simulink model "IMU_dsPIC_30f4012_ComplementaryFilter_20Mips"  (Simulink 7.1)
settings: Solver=FixedStepDiscrete  StartTime=0.0  StopTime=10.0  FixedStep=0.001  RelTol=1e-3
PreLoadFcn:
  | Script_Kalman
undefined symbols (not defined in the file or in its folder): DiscIntNeverNeededParam, gaind, polesd, zerosd
libraries: simulink x10, dsPICdrivers x10
CloseFcn:
  | rtwprivate ssgencode ModelCloseRequest Autopilote_30f4012
settings Model: Creator=Lubin  LastModifiedBy=Lubin
settings OptimizationCC: InlineParams=on  OptimizeModelRefInitCode=on  LifeSpan=1
settings DebuggingCC: SaveWithParameterizedLinksMsg=none  MultiTaskCondExecSysMsg=warning  MultiTaskRateTransMsg=warning
settings HardwareCC: ProdBitPerInt=16  ProdEndianess=LittleEndian  ProdWordSize=16  ProdHWDeviceType=16-bit Generic
settings RTWCC: SystemTargetFile=dspic.tlc  TemplateMakefile=dspic_pic30_gcc.tmf  PostCodeGenCommand=dsPIC_Compile()  Description=Embedded Target for Microchip dsPIC (real-time)  GenerateReport=on  ProcessScript=dspic_make_rtw_hook  IncludeHyperlinkInReport=on  LaunchReport=on  GenerateTraceInfo=on  GenerateTraceReport=on  GenerateTraceReportSl=on  GenerateTraceReportSf=on  GenerateTraceReportEml=on
settings CodeAppCC: IgnoreCustomStorageClasses=off
settings STFCustomTargetCC: ModelReferenceCompliant=off  IncludeMdlTerminateFcn=off  CombineOutputUpdateFcns=on  SuppressErrorStatus=on  ERTCustomFileBanners=on  SupportContinuousTime=off  SupportNonInlinedSFcns=off  SystemTargetFile=dspic.tlc
settings ERTTargetCC: ModelReferenceCompliant=off  CompOptLevelCompliant=off  IncludeMdlTerminateFcn=off  SuppressErrorStatus=on  ERTFirstTimeCompliant=off  ModelStepFunctionPrototypeControlCompliant=off  ExtModeMexFile=ext_serial_win32_comm  InlinedParameterPlacement=NonHierarchical  ERTSrcFileBannerTemplate=dsPIC_code_template.cgt  ERTHdrFileBannerTemplate=dsPIC_code_template.cgt  ERTDataSrcFileTemplate=dsPIC_code_template.cgt  ERTDataHdrFileTemplate=dsPIC_code_template.cgt  ERTCustomFileTemplate=dsPIC_main.tlc
settings CustomProperty: DataType=string  Value=C:\PROGRA~1\MATLAB\R2008a\bin\win32\gmake

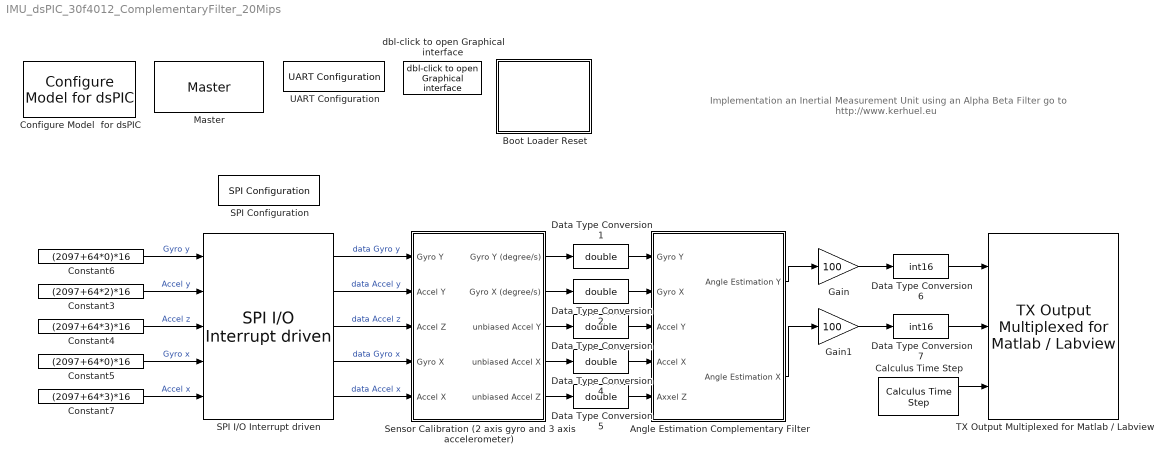
== system IMU_dsPIC_30f4012_ComplementaryFilter_20Mips ==
  note: Implementation an Inertial Measurement Unit using an Alpha Beta Filter
      | go to http://www.kerhuel.eu
  Angle Estimation Complementary Filter : Subsystem
  Boot Loader Reset : Subsystem  AncestorBlock=dsPICdrivers/OTHERS/TinyBld Reset
      mask Display: fprintf('TinyBld\nReset')
  Calculus Time Step : dsPICdrivers/OTHERS/Calculus Time Step  Tag=dsPIC_CalculusTimeStep  SampleTime=-1  PR1chk=on
  Configure Model  for dsPIC : dsPICdrivers/Simulink Configuration/Configure Model  for dsPIC
  Constant3 : Constant  Value=(2097+64*2)*16  VectorParams1D=off  OutDataTypeMode=uint16  OutDataType=sfix(16)  OutScaling=2^0  OutDataTypeStr=uint16  SampleTime=-1
  Constant4 : Constant  Value=(2097+64*3)*16  VectorParams1D=off  OutDataTypeMode=uint16  OutDataType=sfix(16)  OutScaling=2^0  OutDataTypeStr=uint16  SampleTime=-1
  Constant5 : Constant  Value=(2097+64*0)*16  VectorParams1D=off  OutDataTypeMode=uint16  OutDataType=sfix(16)  OutScaling=2^0  OutDataTypeStr=uint16  SampleTime=-1
  Constant6 : Constant  Value=(2097+64*0)*16  VectorParams1D=off  OutDataTypeMode=uint16  OutDataType=sfix(16)  OutScaling=2^0  OutDataTypeStr=uint16  SampleTime=-1
  Constant7 : Constant  Value=(2097+64*3)*16  VectorParams1D=off  OutDataTypeMode=uint16  OutDataType=sfix(16)  OutScaling=2^0  OutDataTypeStr=uint16  SampleTime=-1
  Data Type Conversion{,1..2,4..5} (5 alike) : DataTypeConversion  OutDataTypeMode=double  OutDataType=sfix(16)  OutScaling=2^0  OutDataTypeStr=double
  Data Type Conversion6 : DataTypeConversion  OutDataTypeMode=int16  OutDataType=sfix(16)  OutScaling=2^0  OutDataTypeStr=int16
  Data Type Conversion7 : DataTypeConversion  OutDataTypeMode=int16  OutDataType=sfix(16)  OutScaling=2^0  OutDataTypeStr=int16
  Gain : Gain  Gain=100  ParameterDataType=sfix(16)  ParameterScaling=2^0  OutDataType=sfix(16)  OutScaling=2^0
  Gain1 : Gain  Gain=100  ParameterDataType=sfix(16)  ParameterScaling=2^0  OutDataType=sfix(16)  OutScaling=2^0
  Master : dsPICdrivers/Master  Tag=dsPIC_MASTER  Priority=1  TimeStepType=Timer1  picType=30f4012  fcy=20e6  Quartz_33f=5e6  PLLActive_33f=off  fcyDesired_33f=0  tmr1="[1  19999  0]"  tmr1Info="Time Step : 0.001  ;   Error : 0%  PR1=19999"  tmr2345="[0  0  0  0]"  tmr2345cfg=[-1 -1 -1 -1]  IOautoConf=on  typePort="[ 0   0   0   0   0   0   0   0   0   0   0   0   0   0   0   0   0   0   0   0   0   0   0   0   0   0   0   0   0   0   0   0   0   0   0   0   0   0   0   0   0   0   0   0   0   5   4   0   0   0   0   0   0   0   0   0   0   0   0   0   0   0   0   0   0   0   0  21   0  21   0   0  17   0   0   0   0   0   0   0   0   0   0   0   0   0   0   0   0   0   0   0   0   0   0   0   0   0   0   0   0   0   0   0   0   0   0   0   0   0   0   0 ]"  TRIS="[ 65535  65535  65535  65535  65495  65535  65535 ]"  ADPCFG=0  MasterBusyPort=None  MasterOverloadPort=None  FOSC=XT_PLL8  TempProtection_33f=TEMP_ON  FPBOR=PBOR_OFF  PWRT=PWRT_4  MCLR=MCLR_DIS  PowerSave=off
  SPI Configuration : dsPICdrivers/SPI PORT/SPI Configuration  Tag=dsPIC_config_SPI  Priority=2  ConfigurationTime=At boot time (only once)  OrderingInOutPopup=None  SampleTime=-1  Frame_Enable=0  Frame_Sync=0  SPI=1  MODE=MASTER  USER_SCALER=96  StartEnable=Enable  SDO_EN=on  DATA_LENGTH=16 bits  SS_EN=off  SMP=Middle of bit  CKP=high  CKE=Idle to Active  Status="Mode 1  -    Fsck= Not Available"
  SPI I/O Interrupt driven : dsPICdrivers/SPI PORT/SPI I//O Interrupt driven  Tag=dsPIC_SPI_IO_Interrupt  SPI=1  nbrTrame=5  mode=read once - interrupt re-enable after block execution  Disable=on  DATA_LENGTH=16 bits  OrderingInOutPopup=None  SampleTime=.001  T1CSL=E5  T1CSH=None  T2CSL=E5  T2CSH=None  T3CSL=E5  T3CSH=None  T4CSL=E3  T4CSH=None  T5CSL=E3  T5CSH=None  T6CSL=None  T6CSH=None  T7CSL=None  T7CSH=None  T8CSL=None  T8CSH=None  T9CSL=None  T9CSH=None  T10CSL=None  T10CSH=None  T11CSL=None  T11CSH=None  T12CSL=None  T12CSH=None  T13CSL=None  T13CSH=None  T14CSL=None  T14CSH=None  T15CSL=None  T15CSH=None
  Sensor Calibration (2 axis gyro and 3 axis accelerometer) : Subsystem
  TX Output Multiplexed for Matlab / Labview : dsPICdrivers/Serial PORT/TX Output Multiplexed for Matlab // Labview  Tag=dsPIC_TX_Multiplexed  Priority=5  UART=1  CleverSpreadingChk=on  CleverSpreading=1  CHANNEL=[0 1 2]  CHANNELBLOCKED=[]  CHANNELBLOCKED_BITEWISE=0  Status=OK
  UART Configuration : dsPICdrivers/Serial PORT/UART Configuration  Tag=dsPIC_config_UART  Priority=2  UART=1  proposed_BAUD=115200  ALT_TX_RX=on  InterruptTxWhen=When Transmit Buffer is empty  TXInterruptPri=1  TxBufferSize=32  TXEN=on  InterruptRxWhen=When Receive Buffer is full (contain 4 characters)  RXInterruptPri=1  RxBufferSize=32  BAUD=115200  UxBRG=10  Info="UxBRG = 10   ||  Real Baud : 113636   ||  % error : -1.3573  ||  max 11.3636 Bytes / Step"  RealBaud=0
  dbl-click to open Graphical interface : dsPICdrivers/Serial PORT/dbl-click to open Graphical interface  SystemSampleTime=-1  Nothing=0
  wires:
  Constant6/1 -> SPI I/O Interrupt driven/1  "Gyro y"
  Constant3/1 -> SPI I/O Interrupt driven/2  "Accel y"
  Constant4/1 -> SPI I/O Interrupt driven/3  "Accel z"
  Constant5/1 -> SPI I/O Interrupt driven/4  "Gyro x"
  Constant7/1 -> SPI I/O Interrupt driven/5  "Accel x"
  Gain/1 -> Data Type Conversion6/1
  Gain1/1 -> Data Type Conversion7/1
  Data Type Conversion6/1 -> TX Output Multiplexed for Matlab / Labview/1
  Data Type Conversion7/1 -> TX Output Multiplexed for Matlab / Labview/2
  Calculus Time Step/1 -> TX Output Multiplexed for Matlab / Labview/3
  SPI I/O Interrupt driven/1 -> Sensor Calibration (2 axis gyro and 3 axis accelerometer)/1(Gyro Y)  "data Gyro y"
  SPI I/O Interrupt driven/2 -> Sensor Calibration (2 axis gyro and 3 axis accelerometer)/2(Accel Y)  "data Accel y"
  SPI I/O Interrupt driven/3 -> Sensor Calibration (2 axis gyro and 3 axis accelerometer)/3(Accel Z)  "data Accel z"
  SPI I/O Interrupt driven/4 -> Sensor Calibration (2 axis gyro and 3 axis accelerometer)/4(Gyro X)  "data Gyro x"
  SPI I/O Interrupt driven/5 -> Sensor Calibration (2 axis gyro and 3 axis accelerometer)/5(Accel X)  "data Accel x"
  Data Type Conversion1/1 -> Angle Estimation Complementary Filter/1("Gyro Y ")
  Data Type Conversion2/1 -> Angle Estimation Complementary Filter/2(Gyro X)
  Data Type Conversion/1 -> Angle Estimation Complementary Filter/3(Accel Y)
  Data Type Conversion4/1 -> Angle Estimation Complementary Filter/4(Accel X)
  Data Type Conversion5/1 -> Angle Estimation Complementary Filter/5(Axxel Z)
  Sensor Calibration (2 axis gyro and 3 axis accelerometer)/1(Gyro Y (degree/s)) -> Data Type Conversion1/1
  Sensor Calibration (2 axis gyro and 3 axis accelerometer)/2(Gyro X (degree/s)) -> Data Type Conversion2/1
  Angle Estimation Complementary Filter/1(Angle Estimation Y) -> Gain/1
  Angle Estimation Complementary Filter/2(Angle Estimation X) -> Gain1/1
  Sensor Calibration (2 axis gyro and 3 axis accelerometer)/3(unbiased Accel Y) -> Data Type Conversion/1
  Sensor Calibration (2 axis gyro and 3 axis accelerometer)/4(unbiased Accel X) -> Data Type Conversion4/1
  Sensor Calibration (2 axis gyro and 3 axis accelerometer)/5(unbiased Accel Z) -> Data Type Conversion5/1

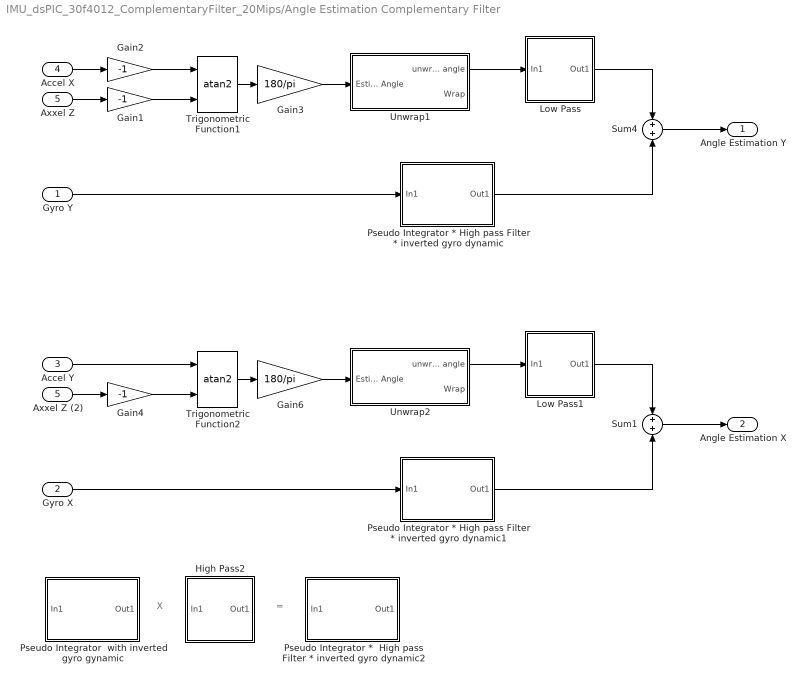
== system IMU_dsPIC_30f4012_ComplementaryFilter_20Mips/Angle Estimation Complementary Filter ==
  note: =
  note: X
  "Gyro Y " : Inport
  Gyro X : Inport  Port=2
  Accel Y : Inport  Port=3
  Accel X : Inport  Port=4
  Axxel Z : Inport  Port=5
  Axxel Z (2) : InportShadow  Port=5  LatchByCopyingInsideSignal=off
  Gain1 : Gain  Gain=-1  ParameterDataType=sfix(16)  ParameterScaling=2^0  OutDataType=sfix(16)  OutScaling=2^0
  Gain2 : Gain  Gain=-1  ParameterDataType=sfix(16)  ParameterScaling=2^0  OutDataType=sfix(16)  OutScaling=2^0
  Gain3 : Gain  Gain=180/pi  ParameterDataType=sfix(16)  ParameterScaling=2^0  OutDataTypeMode=Specify via dialog  OutDataType=float('double')  OutDataTypeStr=float('double')
  Gain4 : Gain  Gain=-1  ParameterDataType=sfix(16)  ParameterScaling=2^0  OutDataType=sfix(16)  OutScaling=2^0
  Gain6 : Gain  Gain=180/pi  ParameterDataType=sfix(16)  ParameterScaling=2^0  OutDataTypeMode=Specify via dialog  OutDataType=float('double')  OutDataTypeStr=float('double')
  High Pass2 : Subsystem  mask(DiscretizedZeroPole){Zeros=[0], Poles=[-.5], Gain=1, AbsTol=auto, SampleTime=.001, method=tustin, Wc=1}
      mask prompts: Zeros "Zeros (enter in s-main:)"; Poles "Poles (enter in s-domain:)"; Gain "Gain (enter in s-domain:)"; AbsTol "Absolute tolerance:"; SampleTime "Sample time:"; Wc "Critical Frequency (Hz):"
      mask help: Continuous mask uses c2d to transform parameters onto the Discrete Zero-Pole block inside.
      mask init:
      | st=SampleTime;
      | if length(st)>1
      |     st=SampleTime(1);
      | end
      | if(st>0)
      |     [zerosd,polesd,gaind] = sldiscutil('disczpk', {st,method,Wc,Zeros,Poles,Gain});
      | end	
      | s = get_param(gcb,'maskvalues');
      | zeross = s{1};
      | poless = s{2};
      | gainss = s{3};
      | %zerosc = eval(zeross);
      | %polesc = eval(poless);
      | %gainsc = eval(gainss);
      | sldiscutil('initzpkmask', st);
      | if(st==0)
      | set_param([gcb '/Zero Pole'], 'AbsoluteTolerance', AbsTol);
      | end
      mask StyleString: edit,edit,edit,edit,edit,popup(zoh|foh|tustin|prewarp|matched),edit
      mask CallbackString: |||||hidecrit|
      mask Display:
      | droots(zeross,poless,gainss)
      | text( 0.5, 1.0, method, 'verticalAlignment','top')
  Low Pass : Subsystem  mask(DiscretizedZeroPole){Zeros=[], Poles=[-.5], Gain=.5, AbsTol=auto, SampleTime=.001, method=tustin, Wc=1}
      mask prompts: Zeros "Zeros (enter in s-main:)"; Poles "Poles (enter in s-domain:)"; Gain "Gain (enter in s-domain:)"; AbsTol "Absolute tolerance:"; SampleTime "Sample time:"; Wc "Critical Frequency (Hz):"
      mask help: Continuous mask uses c2d to transform parameters onto the Discrete Zero-Pole block inside.
      mask init: same as IMU_dsPIC_30f4012_ComplementaryFilter_20Mips/Angle Estimation Complementary Filter/High Pass2
      mask StyleString: edit,edit,edit,edit,edit,popup(zoh|foh|tustin|prewarp|matched),edit
      mask CallbackString: |||||hidecrit|
      mask Display:
      | droots(zeross,poless,gainss)
      | text( 0.5, 1.0, method, 'verticalAlignment','top')
  Low Pass1 : Subsystem  mask(DiscretizedZeroPole){Zeros=[], Poles=[-.5], Gain=.5, AbsTol=auto, SampleTime=.001, method=tustin, Wc=1}
      mask prompts: Zeros "Zeros (enter in s-main:)"; Poles "Poles (enter in s-domain:)"; Gain "Gain (enter in s-domain:)"; AbsTol "Absolute tolerance:"; SampleTime "Sample time:"; Wc "Critical Frequency (Hz):"
      mask help: Continuous mask uses c2d to transform parameters onto the Discrete Zero-Pole block inside.
      mask init: same as IMU_dsPIC_30f4012_ComplementaryFilter_20Mips/Angle Estimation Complementary Filter/High Pass2
      mask StyleString: edit,edit,edit,edit,edit,popup(zoh|foh|tustin|prewarp|matched),edit
      mask CallbackString: |||||hidecrit|
      mask Display:
      | droots(zeross,poless,gainss)
      | text( 0.5, 1.0, method, 'verticalAlignment','top')
  Pseudo Integrator  with inverted gyro gynamic : Subsystem  mask(DiscretizedZeroPole){Zeros=[-314], Poles=[0], Gain=(1/314), AbsTol=auto, SampleTime=.001, method=tustin, Wc=1}
      mask prompts: Zeros "Zeros (enter in s-main:)"; Poles "Poles (enter in s-domain:)"; Gain "Gain (enter in s-domain:)"; AbsTol "Absolute tolerance:"; SampleTime "Sample time:"; Wc "Critical Frequency (Hz):"
      mask help: Continuous mask uses c2d to transform parameters onto the Discrete Zero-Pole block inside.
      mask init: same as IMU_dsPIC_30f4012_ComplementaryFilter_20Mips/Angle Estimation Complementary Filter/High Pass2
      mask StyleString: edit,edit,edit,edit,edit,popup(zoh|foh|tustin|prewarp|matched),edit
      mask CallbackString: |||||hidecrit|
      mask Display:
      | droots(zeross,poless,gainss)
      | text( 0.5, 1.0, method, 'verticalAlignment','top')
  Pseudo Integrator *  High pass Filter * inverted gyro dynamic2 : Subsystem  mask(DiscretizedZeroPole){Zeros=[-314], Poles=[-.5], Gain=(1/314), AbsTol=auto, SampleTime=.001, method=tustin, Wc=1}
      mask prompts: Zeros "Zeros (enter in s-main:)"; Poles "Poles (enter in s-domain:)"; Gain "Gain (enter in s-domain:)"; AbsTol "Absolute tolerance:"; SampleTime "Sample time:"; Wc "Critical Frequency (Hz):"
      mask help: Continuous mask uses c2d to transform parameters onto the Discrete Zero-Pole block inside.
      mask init: same as IMU_dsPIC_30f4012_ComplementaryFilter_20Mips/Angle Estimation Complementary Filter/High Pass2
      mask StyleString: edit,edit,edit,edit,edit,popup(zoh|foh|tustin|prewarp|matched),edit
      mask CallbackString: |||||hidecrit|
      mask Display:
      | droots(zeross,poless,gainss)
      | text( 0.5, 1.0, method, 'verticalAlignment','top')
  Pseudo Integrator * High pass Filter * inverted gyro dynamic : Subsystem  mask(DiscretizedZeroPole){Zeros=[-314], Poles=[-.5], Gain=(1/314), AbsTol=auto, SampleTime=.001, method=tustin, Wc=1}
      mask prompts: Zeros "Zeros (enter in s-main:)"; Poles "Poles (enter in s-domain:)"; Gain "Gain (enter in s-domain:)"; AbsTol "Absolute tolerance:"; SampleTime "Sample time:"; Wc "Critical Frequency (Hz):"
      mask help: Continuous mask uses c2d to transform parameters onto the Discrete Zero-Pole block inside.
      mask init: same as IMU_dsPIC_30f4012_ComplementaryFilter_20Mips/Angle Estimation Complementary Filter/High Pass2
      mask StyleString: edit,edit,edit,edit,edit,popup(zoh|foh|tustin|prewarp|matched),edit
      mask CallbackString: |||||hidecrit|
      mask Display:
      | droots(zeross,poless,gainss)
      | text( 0.5, 1.0, method, 'verticalAlignment','top')
  Pseudo Integrator * High pass Filter * inverted gyro dynamic1 : Subsystem  mask(DiscretizedZeroPole){Zeros=[-314], Poles=[-.5], Gain=(1/314), AbsTol=auto, SampleTime=.001, method=tustin, Wc=1}
      mask prompts: Zeros "Zeros (enter in s-main:)"; Poles "Poles (enter in s-domain:)"; Gain "Gain (enter in s-domain:)"; AbsTol "Absolute tolerance:"; SampleTime "Sample time:"; Wc "Critical Frequency (Hz):"
      mask help: Continuous mask uses c2d to transform parameters onto the Discrete Zero-Pole block inside.
      mask init: same as IMU_dsPIC_30f4012_ComplementaryFilter_20Mips/Angle Estimation Complementary Filter/High Pass2
      mask StyleString: edit,edit,edit,edit,edit,popup(zoh|foh|tustin|prewarp|matched),edit
      mask CallbackString: |||||hidecrit|
      mask Display:
      | droots(zeross,poless,gainss)
      | text( 0.5, 1.0, method, 'verticalAlignment','top')
  Sum1 : Sum  OutDataType=sfix(16)  OutScaling=2^0  SaturateOnIntegerOverflow=on
  Sum4 : Sum  OutDataType=sfix(16)  OutScaling=2^0  SaturateOnIntegerOverflow=on
  Trigonometric Function1 : Trigonometry  Operator=atan2  OutputSignalType=real
  Trigonometric Function2 : Trigonometry  Operator=atan2  OutputSignalType=real
  Unwrap1 : Subsystem
  Unwrap2 : Subsystem
  Angle Estimation Y : Outport
  Angle Estimation X : Outport  Port=2
  wires:
  Pseudo Integrator * High pass Filter * inverted gyro dynamic/1(Out1) -> Sum4/2
  Pseudo Integrator * High pass Filter * inverted gyro dynamic1/1(Out1) -> Sum1/2
  Low Pass/1(Out1) -> Sum4/1
  Accel X/1 -> Gain2/1
  Axxel Z/1 -> Gain1/1
  Sum4/1 -> Angle Estimation Y/1
  "Gyro Y "/1 -> Pseudo Integrator * High pass Filter * inverted gyro dynamic/1(In1)
  Gain2/1 -> Trigonometric Function1/1
  Gain1/1 -> Trigonometric Function1/2
  Trigonometric Function1/1 -> Gain3/1
  Gain3/1 -> Unwrap1/1(Estimated Angle)
  Unwrap1/1(unwrap angle) -> Low Pass/1(In1)
  Low Pass1/1(Out1) -> Sum1/1
  Accel Y/1 -> Trigonometric Function2/1
  Axxel Z (2)/1 -> Gain4/1
  Sum1/1 -> Angle Estimation X/1
  Gyro X/1 -> Pseudo Integrator * High pass Filter * inverted gyro dynamic1/1(In1)
  Gain4/1 -> Trigonometric Function2/2
  Trigonometric Function2/1 -> Gain6/1
  Gain6/1 -> Unwrap2/1(Estimated Angle)
  Unwrap2/1(unwrap angle) -> Low Pass1/1(In1)

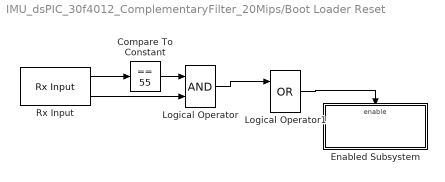
== system IMU_dsPIC_30f4012_ComplementaryFilter_20Mips/Boot Loader Reset ==
  Compare To Constant : simulink/Logic and Bit Operations/Compare To Constant  SystemSampleTime=-1  relop===  const=55  LogicOutDataTypeMode=boolean  ZeroCross=off
  Enabled Subsystem : Subsystem  TreatAsAtomicUnit=on
  Logical Operator : Logic  AllPortsSameDT=off  OutDataTypeMode=boolean  OutDataTypeStr=boolean
  Logical Operator1 : Logic  Operator=OR  AllPortsSameDT=off  OutDataTypeMode=boolean  OutDataTypeStr=boolean
  Rx Input : dsPICdrivers/Serial PORT/Rx Input  Tag=dsPIC_RX  Priority=5  UART=1  SampleTime=.01  BlockingFctChk=off  OutputDefault=0  IsPresentFlagChk=on
  wires:
  Rx Input/1 -> Compare To Constant/1
  Compare To Constant/1 -> Logical Operator/1
  Rx Input/2 -> Logical Operator/2
  Logical Operator/1 -> Logical Operator1/1
  Logical Operator1/1 -> Enabled Subsystem/Enable

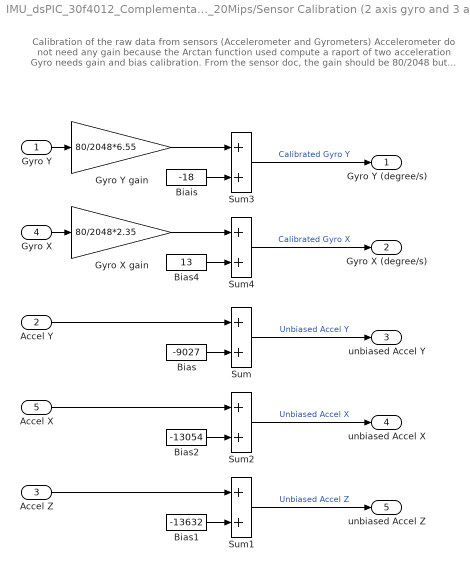
== system IMU_dsPIC_30f4012_ComplementaryFilter_20Mips/Sensor Calibration (2 axis gyro and 3 axis accelerometer) ==
  note: Calibration of the raw data from sensors (Accelerometer and Gyrometers)
      | Accelerometer do not need any gain because the Arctan function used compute a raport of two acceleration
      | Gyro needs gain and bias calibration. From the sensor doc, the gain should be 80/2048 but...
  Gyro Y : Inport
  Accel Y : Inport  Port=2
  Accel Z : Inport  Port=3
  Gyro X : Inport  Port=4
  Accel X : Inport  Port=5
  "Biais " : Constant  Value=-18  OutDataType=sfix(16)  OutScaling=2^0
  Bias : Constant  Value=-9027  OutDataType=sfix(16)  OutScaling=2^0
  Bias1 : Constant  Value=-13632  OutDataType=sfix(16)  OutScaling=2^0
  Bias2 : Constant  Value=-13054  OutDataType=sfix(16)  OutScaling=2^0
  Bias4 : Constant  Value=13  OutDataType=sfix(16)  OutScaling=2^0
  Gyro X gain : Gain  Gain=80/2048*2.35  ParameterDataType=sfix(16)  ParameterScaling=2^0  OutDataTypeMode=Specify via dialog  OutDataType=float('double')  OutDataTypeStr=float('double')
  Gyro Y gain : Gain  Gain=80/2048*6.55  ParameterDataType=sfix(16)  ParameterScaling=2^0  OutDataTypeMode=Specify via dialog  OutDataType=float('double')  OutDataTypeStr=float('double')
  Sum{,1..4} (5 alike) : Sum  OutDataType=sfix(16)  OutScaling=2^0
  Gyro Y (degree/s) : Outport
  Gyro X (degree/s) : Outport  Port=2
  unbiased Accel Y : Outport  Port=3
  unbiased Accel X : Outport  Port=4
  unbiased Accel Z : Outport  Port=5
  wires:
  Bias4/1 -> Sum4/2
  Sum4/1 -> Gyro X (degree/s)/1  "Calibrated Gyro X"
  Gyro X gain/1 -> Sum4/1
  "Biais "/1 -> Sum3/2
  Sum3/1 -> Gyro Y (degree/s)/1  "Calibrated Gyro Y"
  Gyro Y gain/1 -> Sum3/1
  Sum2/1 -> unbiased Accel X/1  "Unbiased Accel X"
  Accel X/1 -> Sum2/1
  Gyro X/1 -> Gyro X gain/1
  Sum1/1 -> unbiased Accel Z/1  "Unbiased Accel Z"
  Accel Z/1 -> Sum1/1
  Sum/1 -> unbiased Accel Y/1  "Unbiased Accel Y"
  Accel Y/1 -> Sum/1
  Gyro Y/1 -> Gyro Y gain/1
  Bias2/1 -> Sum2/2
  Bias1/1 -> Sum1/2
  Bias/1 -> Sum/2

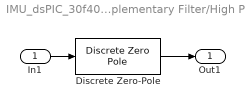
== system IMU_dsPIC_30f4012_ComplementaryFilter_20Mips/Angle Estimation Complementary Filter/High Pass2 ==
  In1 : Inport  OutDataType=sfix(16)  OutScaling=2^0
  Discrete Zero-Pole : DiscreteZeroPole  Zeros=zerosd  Poles=polesd  Gain=gaind  SampleTime=SampleTime
  Out1 : Outport  OutDataType=sfix(16)  OutScaling=2^0
  wires:
  In1/1 -> Discrete Zero-Pole/1
  Discrete Zero-Pole/1 -> Out1/1

== system IMU_dsPIC_30f4012_ComplementaryFilter_20Mips/Angle Estimation Complementary Filter/Low Pass ==
  In1 : Inport  OutDataType=sfix(16)  OutScaling=2^0
  Discrete Zero-Pole : DiscreteZeroPole  Zeros=zerosd  Poles=polesd  Gain=gaind  SampleTime=SampleTime
  Out1 : Outport  OutDataType=sfix(16)  OutScaling=2^0
  wires:
  In1/1 -> Discrete Zero-Pole/1
  Discrete Zero-Pole/1 -> Out1/1

== system IMU_dsPIC_30f4012_ComplementaryFilter_20Mips/Angle Estimation Complementary Filter/Low Pass1 ==
  In1 : Inport  OutDataType=sfix(16)  OutScaling=2^0
  Discrete Zero-Pole : DiscreteZeroPole  Zeros=zerosd  Poles=polesd  Gain=gaind  SampleTime=SampleTime
  Out1 : Outport  OutDataType=sfix(16)  OutScaling=2^0
  wires:
  Discrete Zero-Pole/1 -> Out1/1
  In1/1 -> Discrete Zero-Pole/1

== system IMU_dsPIC_30f4012_ComplementaryFilter_20Mips/Angle Estimation Complementary Filter/Pseudo Integrator  with inverted gyro gynamic ==
  In1 : Inport  OutDataType=sfix(16)  OutScaling=2^0
  Discrete Zero-Pole : DiscreteZeroPole  Zeros=zerosd  Poles=polesd  Gain=gaind  SampleTime=SampleTime
  Out1 : Outport  OutDataType=sfix(16)  OutScaling=2^0
  wires:
  In1/1 -> Discrete Zero-Pole/1
  Discrete Zero-Pole/1 -> Out1/1

== system IMU_dsPIC_30f4012_ComplementaryFilter_20Mips/Angle Estimation Complementary Filter/Pseudo Integrator *  High pass Filter * inverted gyro dynamic2 ==
  In1 : Inport  OutDataType=sfix(16)  OutScaling=2^0
  Discrete Zero-Pole : DiscreteZeroPole  Zeros=zerosd  Poles=polesd  Gain=gaind  SampleTime=SampleTime
  Out1 : Outport  OutDataType=sfix(16)  OutScaling=2^0
  wires:
  In1/1 -> Discrete Zero-Pole/1
  Discrete Zero-Pole/1 -> Out1/1

== system IMU_dsPIC_30f4012_ComplementaryFilter_20Mips/Angle Estimation Complementary Filter/Pseudo Integrator * High pass Filter * inverted gyro dynamic ==
  In1 : Inport  OutDataType=sfix(16)  OutScaling=2^0
  Discrete Zero-Pole : DiscreteZeroPole  Zeros=zerosd  Poles=polesd  Gain=gaind  SampleTime=SampleTime
  Out1 : Outport  OutDataType=sfix(16)  OutScaling=2^0
  wires:
  In1/1 -> Discrete Zero-Pole/1
  Discrete Zero-Pole/1 -> Out1/1

== system IMU_dsPIC_30f4012_ComplementaryFilter_20Mips/Angle Estimation Complementary Filter/Pseudo Integrator * High pass Filter * inverted gyro dynamic1 ==
  In1 : Inport  OutDataType=sfix(16)  OutScaling=2^0
  Discrete Zero-Pole : DiscreteZeroPole  Zeros=zerosd  Poles=polesd  Gain=gaind  SampleTime=SampleTime
  Out1 : Outport  OutDataType=sfix(16)  OutScaling=2^0
  wires:
  Discrete Zero-Pole/1 -> Out1/1
  In1/1 -> Discrete Zero-Pole/1

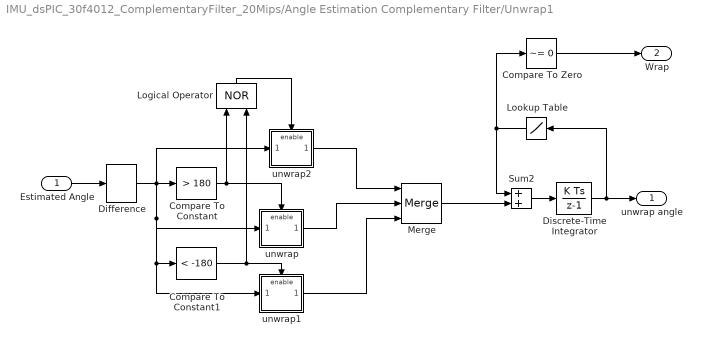
== system IMU_dsPIC_30f4012_ComplementaryFilter_20Mips/Angle Estimation Complementary Filter/Unwrap1 ==
  Estimated Angle : Inport
  Compare To Constant : simulink/Logic and Bit Operations/Compare To Constant  SystemSampleTime=-1  relop=>  const=180  LogicOutDataTypeMode=uint8  ZeroCross=off
  Compare To Constant1 : simulink/Logic and Bit Operations/Compare To Constant  SystemSampleTime=-1  relop=<  const=-180  LogicOutDataTypeMode=uint8  ZeroCross=off
  Compare To Zero : simulink/Logic and Bit Operations/Compare To Zero  SystemSampleTime=-1  relop=~=  LogicOutDataTypeMode=uint8  ZeroCross=off
  Difference : simulink/Discrete/Difference  SystemSampleTime=-1  ICPrevInput=0.0  OutMin=[]  OutMax=[]  OutDataType=sfix(16)  OutScaling=2^-10  DoSatur=off
  Discrete-Time Integrator : DiscreteIntegrator  gainval=1000  SampleTime=-1  OutDataType=sfix(16)  OutScaling=2^0  ICPrevOutput=DiscIntNeverNeededParam  ICPrevScaledInput=DiscIntNeverNeededParam
  Logical Operator : Logic  Orientation=up  Operator=NOR  AllPortsSameDT=off  OutDataTypeMode=boolean  OutDataTypeStr=boolean
  Lookup Table : Lookup  Orientation=left  InputValues=[-500 -195 195]  Table=[+360 0 -360]  LookUpMeth=Use Input Below  OutDataType=sfix(16)  OutScaling=2^0
  Merge : Merge  Inputs=3
  Sum2 : Sum  OutDataType=sfix(16)  OutScaling=2^0
  unwrap : Subsystem  TreatAsAtomicUnit=on
  unwrap1 : Subsystem  TreatAsAtomicUnit=on
  unwrap2 : Subsystem  TreatAsAtomicUnit=on
  unwrap angle : Outport
  Wrap : Outport  Port=2
  wires:
  Compare To Zero/1 -> Wrap/1
  Lookup Table/1 -> Compare To Zero/1, Sum2/1
  Merge/1 -> Sum2/2
  Sum2/1 -> Discrete-Time Integrator/1
  Difference/1 -> Compare To Constant/1, unwrap/1(In1), Compare To Constant1/1, unwrap1/1(In1), unwrap2/1(In1)
  Compare To Constant/1 -> Logical Operator/1, unwrap/Enable
  Compare To Constant1/1 -> unwrap1/Enable, Logical Operator/2
  Logical Operator/1 -> unwrap2/Enable
  unwrap2/1(Out1) -> Merge/1
  unwrap/1(Out1) -> Merge/2
  unwrap1/1(Out1) -> Merge/3
  Estimated Angle/1 -> Difference/1
  Discrete-Time Integrator/1 -> Lookup Table/1, unwrap angle/1

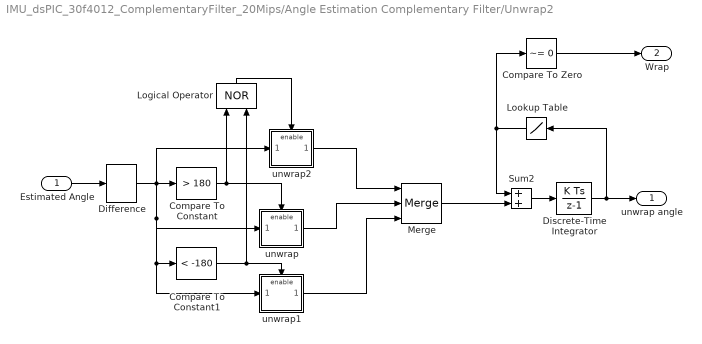
== system IMU_dsPIC_30f4012_ComplementaryFilter_20Mips/Angle Estimation Complementary Filter/Unwrap2 ==
  Estimated Angle : Inport
  Compare To Constant : simulink/Logic and Bit Operations/Compare To Constant  SystemSampleTime=-1  relop=>  const=180  LogicOutDataTypeMode=uint8  ZeroCross=off
  Compare To Constant1 : simulink/Logic and Bit Operations/Compare To Constant  SystemSampleTime=-1  relop=<  const=-180  LogicOutDataTypeMode=uint8  ZeroCross=off
  Compare To Zero : simulink/Logic and Bit Operations/Compare To Zero  SystemSampleTime=-1  relop=~=  LogicOutDataTypeMode=uint8  ZeroCross=off
  Difference : simulink/Discrete/Difference  SystemSampleTime=-1  ICPrevInput=0.0  OutMin=[]  OutMax=[]  OutDataType=sfix(16)  OutScaling=2^-10  DoSatur=off
  Discrete-Time Integrator : DiscreteIntegrator  gainval=1000  SampleTime=-1  OutDataType=sfix(16)  OutScaling=2^0  ICPrevOutput=DiscIntNeverNeededParam  ICPrevScaledInput=DiscIntNeverNeededParam
  Logical Operator : Logic  Orientation=up  Operator=NOR  AllPortsSameDT=off  OutDataTypeMode=boolean  OutDataTypeStr=boolean
  Lookup Table : Lookup  Orientation=left  InputValues=[-500 -195 195]  Table=[+360 0 -360]  LookUpMeth=Use Input Below  OutDataType=sfix(16)  OutScaling=2^0
  Merge : Merge  Inputs=3
  Sum2 : Sum  OutDataType=sfix(16)  OutScaling=2^0
  unwrap : Subsystem  TreatAsAtomicUnit=on
  unwrap1 : Subsystem  TreatAsAtomicUnit=on
  unwrap2 : Subsystem  TreatAsAtomicUnit=on
  unwrap angle : Outport
  Wrap : Outport  Port=2
  wires:
  Discrete-Time Integrator/1 -> unwrap angle/1, Lookup Table/1
  Estimated Angle/1 -> Difference/1
  unwrap1/1(Out1) -> Merge/3
  unwrap/1(Out1) -> Merge/2
  unwrap2/1(Out1) -> Merge/1
  Logical Operator/1 -> unwrap2/Enable
  Compare To Constant1/1 -> Logical Operator/2, unwrap1/Enable
  Compare To Constant/1 -> unwrap/Enable, Logical Operator/1
  Difference/1 -> unwrap2/1(In1), unwrap1/1(In1), Compare To Constant1/1, unwrap/1(In1), Compare To Constant/1
  Sum2/1 -> Discrete-Time Integrator/1
  Merge/1 -> Sum2/2
  Lookup Table/1 -> Sum2/1, Compare To Zero/1
  Compare To Zero/1 -> Wrap/1

== system IMU_dsPIC_30f4012_ComplementaryFilter_20Mips/Boot Loader Reset/Enabled Subsystem ==
  Enable : EnablePort
  While Iterator Subsystem : Subsystem  TreatAsAtomicUnit=on

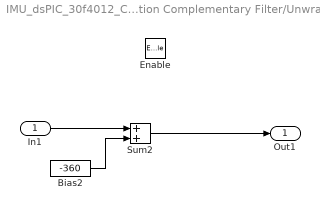
== system IMU_dsPIC_30f4012_ComplementaryFilter_20Mips/Angle Estimation Complementary Filter/Unwrap1/unwrap ==
  In1 : Inport  OutDataType=sfix(16)  OutScaling=2^0
  Enable : EnablePort
  Bias2 : Constant  Value=-360  OutDataType=sfix(16)  OutScaling=2^0
  Sum2 : Sum  OutDataType=sfix(16)  OutScaling=2^0
  Out1 : Outport  OutDataType=sfix(16)  OutScaling=2^0
  wires:
  In1/1 -> Sum2/1
  Sum2/1 -> Out1/1
  Bias2/1 -> Sum2/2

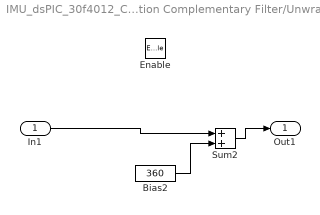
== system IMU_dsPIC_30f4012_ComplementaryFilter_20Mips/Angle Estimation Complementary Filter/Unwrap1/unwrap1 ==
  In1 : Inport  OutDataType=sfix(16)  OutScaling=2^0
  Enable : EnablePort
  Bias2 : Constant  Value=360  OutDataType=sfix(16)  OutScaling=2^0
  Sum2 : Sum  OutDataType=sfix(16)  OutScaling=2^0
  Out1 : Outport  OutDataType=sfix(16)  OutScaling=2^0
  wires:
  In1/1 -> Sum2/1
  Bias2/1 -> Sum2/2
  Sum2/1 -> Out1/1

== system IMU_dsPIC_30f4012_ComplementaryFilter_20Mips/Angle Estimation Complementary Filter/Unwrap1/unwrap2 ==
  In1 : Inport  OutDataType=sfix(16)  OutScaling=2^0
  Enable : EnablePort
  Out1 : Outport  OutDataType=sfix(16)  OutScaling=2^0
  wires:
  In1/1 -> Out1/1

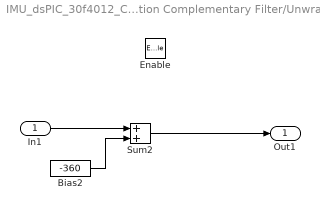
== system IMU_dsPIC_30f4012_ComplementaryFilter_20Mips/Angle Estimation Complementary Filter/Unwrap2/unwrap ==
  In1 : Inport  OutDataType=sfix(16)  OutScaling=2^0
  Enable : EnablePort
  Bias2 : Constant  Value=-360  OutDataType=sfix(16)  OutScaling=2^0
  Sum2 : Sum  OutDataType=sfix(16)  OutScaling=2^0
  Out1 : Outport  OutDataType=sfix(16)  OutScaling=2^0
  wires:
  Bias2/1 -> Sum2/2
  Sum2/1 -> Out1/1
  In1/1 -> Sum2/1

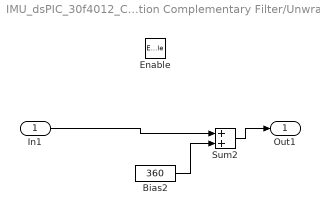
== system IMU_dsPIC_30f4012_ComplementaryFilter_20Mips/Angle Estimation Complementary Filter/Unwrap2/unwrap1 ==
  In1 : Inport  OutDataType=sfix(16)  OutScaling=2^0
  Enable : EnablePort
  Bias2 : Constant  Value=360  OutDataType=sfix(16)  OutScaling=2^0
  Sum2 : Sum  OutDataType=sfix(16)  OutScaling=2^0
  Out1 : Outport  OutDataType=sfix(16)  OutScaling=2^0
  wires:
  Sum2/1 -> Out1/1
  Bias2/1 -> Sum2/2
  In1/1 -> Sum2/1

== system IMU_dsPIC_30f4012_ComplementaryFilter_20Mips/Angle Estimation Complementary Filter/Unwrap2/unwrap2 ==
  In1 : Inport  OutDataType=sfix(16)  OutScaling=2^0
  Enable : EnablePort
  Out1 : Outport  OutDataType=sfix(16)  OutScaling=2^0
  wires:
  In1/1 -> Out1/1

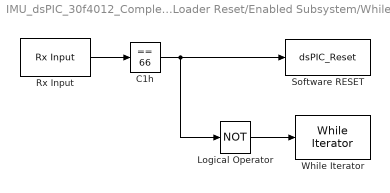
== system IMU_dsPIC_30f4012_ComplementaryFilter_20Mips/Boot Loader Reset/Enabled Subsystem/While Iterator Subsystem ==
  C1h : simulink/Logic and Bit Operations/Compare To Constant  SystemSampleTime=-1  relop===  const=66  LogicOutDataTypeMode=boolean  ZeroCross=off
  Logical Operator : Logic  Operator=NOT  AllPortsSameDT=off  OutDataTypeMode=boolean  OutDataTypeStr=boolean
  Rx Input : dsPICdrivers/Serial PORT/Rx Input  Tag=dsPIC_RX  Priority=5  UART=1  SampleTime=-1  BlockingFctChk=on  OutputDefault=0  IsPresentFlagChk=off
  Software RESET : S-Function  Tag=dsPIC_Reset  FunctionName=dsPIC_Reset  EnableBusSupport=off
      mask Description: Reset the microcontroller when input is different from 0
      mask Display:
      | fprintf('Reset');
      | port_label('input', 1 ,'~=0');
  While Iterator : WhileIterator  MaxIters=-1  WhileBlockType=do-while  ResetStates=reset
  wires:
  Logical Operator/1 -> While Iterator/1
  Rx Input/1 -> C1h/1
  C1h/1 -> Software RESET/1, Logical Operator/1
